simulink model "regulator_lim"  (R2019a)
settings: Solver=FixedStepAuto  StartTime=0.0  StopTime=20  FixedStep=sT  RelTol=1e-3
InitFcn:
  | param;
values from neighbouring files (symbols this model uses):
  A = [0 1; w^2 0]    [continus.m]    (also in discrete.m = [0 1; omega^2 0]; param.m = [0 1; omega^2 0]; param2.m = [0 1; omega^2 0]; param_kf.m)
  B = [0; -w^2]    [continus.m]    (also in discrete.m = [0; -omega^2]; param.m = [0; -omega^2]; param2.m = [0; -omega^2]; param_kf.m)
  C = eye(2)    [discrete.m]    (also in param.m; param2.m; param_kf.m = [w^2 0]; test0.m)
  D = [0 0]'    [discrete.m]    (also in param.m; param2.m; param_kf.m = -w^2; test0.m)
  inix = [0.00 0.0]'    [param.m]    (also in param2.m = [0.05 0.0]'; param_kf.m = [0.0 0.0]')
  iniXzmax = 0.07    [param.m]    (also in param2.m; param_kf.m)
  iniXzmin = -0.07    [param.m]    (also in param2.m; param_kf.m)
  K = [k1 k2]    [continus.m]    (also in discrete.m = -place(A, B, [q1 q2]); param.m; param2.m = dlqr(A,B,Q,H); param_kf.m = -place(A, B, [q1 q2]))
  omega = sqrt(g/zc)    [discrete.m]    (also in param.m; param2.m; test0.m)
  q2 = -0.00005    (= -5e-05)    [discrete.m]    (also in param.m = -0.6; param2.m = -0.5; param_kf.m = -0.5; test0.m = -8-4j)
  sT = 0.01    [discrete.m]    (also in param.m; param2.m; param_kf.m; test0.m)
settings Model: Creator=hideaki  LastModifiedBy=hideaki

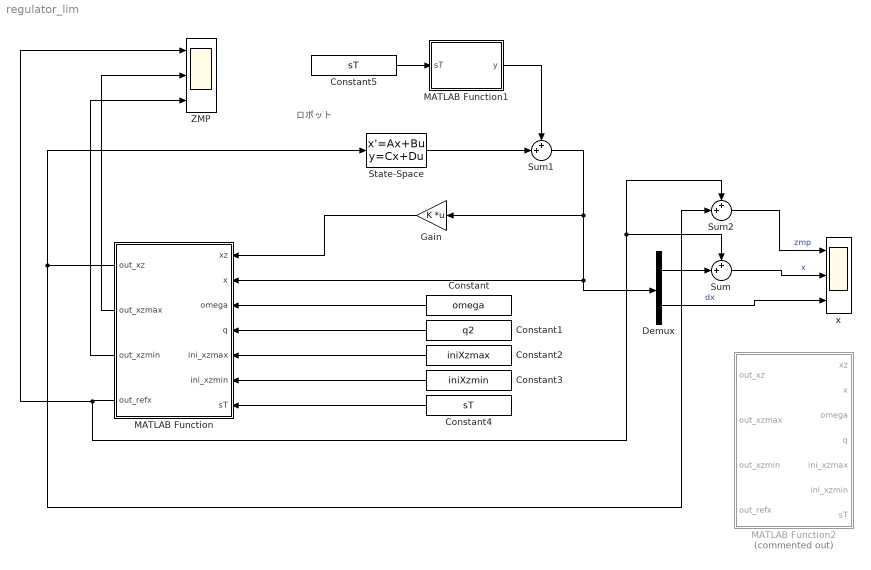
== system regulator_lim ==
  note: ロボット
  Constant : Constant  Value=omega
  Constant1 : Constant  Value=q2
  Constant2 : Constant  Value=iniXzmax
  Constant3 : Constant  Value=iniXzmin
  Constant4 : Constant  Value=sT
  Constant5 : Constant  Value=sT
  Demux : Demux  Outputs=2
  Gain : Gain  Gain=K  Multiplication=Matrix(K*u)
  MATLAB Function : MATLAB Function  TreatAsAtomicUnit=on  SystemSampleTime=sT
  MATLAB Function1 : MATLAB Function  TreatAsAtomicUnit=on
  MATLAB Function2 : MATLAB Function  Commented=on  TreatAsAtomicUnit=on  SystemSampleTime=sT
  State-Space : StateSpace  A=A  B=B  C=C  D=D  InitialCondition=inix
  Sum : Sum  Inputs=++|
  Sum1 : Sum  Inputs=++|
  Sum2 : Sum  Inputs=++|
  ZMP : Scope  NumInputPorts=3
  x : Scope  NumInputPorts=3
  wires:
  Sum1/1 -> Demux/1, MATLAB Function/2(x), Gain/1
  Gain/1 -> MATLAB Function/1(xz)
  MATLAB Function/1(out_xz) -> State-Space/1, Sum2/2
  MATLAB Function/2(out_xzmax) -> ZMP/2
  MATLAB Function/3(out_xzmin) -> ZMP/3
  Constant/1 -> MATLAB Function/3(omega)
  Constant1/1 -> MATLAB Function/4(q)
  Constant2/1 -> MATLAB Function/5(ini_xzmax)
  Constant3/1 -> MATLAB Function/6(ini_xzmin)
  Constant4/1 -> MATLAB Function/7(sT)
  Demux/1 -> Sum/2
  MATLAB Function/4(out_refx) -> ZMP/1, Sum2/1, Sum/1
  Sum/1 -> x/2  "x"
  State-Space/1 -> Sum1/2
  MATLAB Function1/1(y) -> Sum1/1
  Constant5/1 -> MATLAB Function1/1(sT)
  Demux/2 -> x/3  "dx"
  Sum2/1 -> x/1  "zmp"

== matlab function regulator_lim/MATLAB Function1 ==
  data: y output; sT input
function y = nois(sT)
    
    y = zeros(2,1);
    persistent tCnt;
    if isempty(tCnt)
        tCnt = 0;
    end
    
    if (tCnt >= 1 && tCnt <= 1.1) 
        y(2) = -0.4;
    end
    
    tCnt = tCnt + sT;
end

== matlab function regulator_lim/MATLAB Function ==
  data: xz input; out_xz output; x input; out_xzmax output; out_xzmin output; omega input; q input; ini_xzmax input; ini_xzmin input; sT input; out_refx output
%%
% ZMPの出力
% 
%
function [out_xz,out_xzmax,out_xzmin,out_refx] = fcn(xz,x,omega,q,ini_xzmax,ini_xzmin,sT)
    
    persistent tCnt;
    
    %重心の参照位置（目標値）
    persistent refx;
    %実際の支持領域
    persistent xzmax;
    persistent xzmin;
    %refxを基準にした支持領域
    persistent Xzmax;
    persistent Xzmin;
    
    %以下、離床時に計算されて、着地まで保持した後に着地で出力
    persistent s_xz;
    persistent landing;
    persistent s_xzmax;
    persistent s_xzmin;
    persistent s_refx;
    
    %refxを基準にした重心の位置
    X = 0;
    %refxを基準にした重心の速度（速度はどこを基準にしても変わらない）
    dX = 0;
    %refxを基準にしたZMP
    Xz = 0;
    
    if isempty(tCnt)
        tCnt = 0;
        xzmax = ini_xzmax;
        xzmin = ini_xzmin;
        s_xz = xz;
        landing = 0;
        s_xzmax = xzmax;
        s_xzmin = xzmin;
        s_refx = 0;
        refx = getRefx(xzmax,xzmin);
        Xzmax = xzmax - refx;
        Xzmin = xzmin - refx;
    end
    
    X = x(1) - refx;
    dX = x(2);
    Xz = xz -refx;
    
    %立位化安定領域から外れた（xzmin以下）
    if (X+(dX/omega) <= Xzmin) 
        %両足支持
        %支持領域を広げるために、まずは片足支持に移行する
        %if (xzmax == 0.07 && xzmin == -0.07 && landing == 0)
            %強制的に支持領域を狭める（傾いてる方の足を上げる）
            xzmin = 0.01;
            refx = getRefx(xzmax,xzmin);
            %実際のZMP
            s_xz = Xz +refx; 
            %両足支持の場合は離床なのですぐに反映する
            xz = s_xz;
            
            %重心の参照位置は、この時点では変えない
            refx = 0;
            
            %refxを基準としたZMP
            Xz = (1+q)*(X+(dX/omega));
            Xzmin = Xz;
            s_xzmin = Xzmin + refx;
            s_refx = getRefx(xzmax,s_xzmin);
            %実際のZMP（片足支持の場合は着地までに0.6秒かかる）
            s_xz = Xz + refx;
            %着地まで待ち
            tCnt = 0;
            landing = 1;
        %end
    end
    
    %着地
    if (tCnt >= 0.6 && landing == 1) 
        xzmin = s_xzmin;
        refx = s_refx;
        xz = s_xz;
        landing = 2;
    %elseif (landing == 1)
        %実際のロボットでは、ここで両足の中心を重心の参照位置にする（ロボットの遊脚は毎時刻動いている）
        %refx = refx - (abs(s_xzmin) + abs(xzmax))/0.6;
        
    end
    
    
    
    %支持領域の拘束
    if (xz > xzmax) 
        out_xz = xzmax;      
    elseif (xz < xzmin)
        out_xz = xzmin;   
    else
        out_xz = xz;
    end
    
    out_xzmax = xzmax;
    out_xzmin = xzmin;
    out_refx = refx;
    
    tCnt = tCnt + sT;
end

%%
% 重心の参照位置
%
function refx = getRefx(xzmax,xzmin) 
    
    if (0 > xzmax)
        refx = xzmax;
    elseif (0 < xzmin) 
        refx = xzmin;
    else
        refx = (xzmax+xzmin)/2;
    end
    
end

== matlab function regulator_lim/MATLAB Function2 ==
  data: xz input; out_xz output; x input; out_xzmax output; out_xzmin output; omega input; q input; ini_xzmax input; ini_xzmin input; sT input; out_refx output
%%
% ZMPの出力
% 
%
function [out_xz,out_xzmax,out_xzmin,out_refx] = fcn(xz,x,omega,q,ini_xzmax,ini_xzmin,sT)
    
    persistent tCnt;
    
    %重心の参照位置（目標値）
    persistent refx;
    %実際の支持領域
    persistent xzmax;
    persistent xzmin;
    %refxを基準にした支持領域
    persistent Xzmax;
    persistent Xzmin;
    
    %以下、離床時に計算されて、着地まで保持した後に着地で出力
    persistent s_xz;
    persistent landing;
    persistent s_xzmax;
    persistent s_xzmin;
    persistent s_refx;
    
    %refxを基準にした重心の位置
    X = 0;
    %refxを基準にした重心の速度（速度はどこを基準にしても変わらない）
    dX = 0;
    %refxを基準にしたZMP
    Xz = 0;
    
    if isempty(tCnt)
        tCnt = 0;
        xzmax = ini_xzmax;
        xzmin = ini_xzmin;
        s_xz = xz;
        landing = 0;
        s_xzmax = xzmax;
        s_xzmin = xzmin;
        s_refx = 0;
        refx = getRefx(xzmax,xzmin);
        Xzmax = xzmax - refx;
        Xzmin = xzmin - refx;
    end
    
    X = x(1) - refx;
    dX = x(2);
    Xz = xz -refx;
    
    %立位化安定領域から外れた（xzmin以下）
    if (X+(dX/omega) <= Xzmin) 
        %両足支持
        %支持領域を広げるために、まずは片足支持に移行する
        %if (xzmax == 0.07 && xzmin == -0.07 && landing == 0)
            %強制的に支持領域を狭める（傾いてる方の足を上げる）
            xzmin = 0.01;
            refx = getRefx(xzmax,xzmin);
            %実際のZMP
            s_xz = Xz +refx; 
            %両足支持の場合は離床なのですぐに反映する
            xz = s_xz;
            
            %重心の参照位置は、この時点では変えない
            refx = 0;
            
            %refxを基準としたZMP
            Xz = (1+q)*(X+(dX/omega));
            Xzmin = Xz;
            s_xzmin = Xzmin + refx;
            s_refx = getRefx(xzmax,s_xzmin);
            %実際のZMP（片足支持の場合は着地までに0.6秒かかる）
            s_xz = Xz + refx;
            %着地まで待ち
            tCnt = 0;
            landing = 1;
        %end
    end
    
    %着地
    if (tCnt >= 0.6 && landing == 1) 
        xzmin = s_xzmin;
        refx = s_refx;
        xz = s_xz;
        landing = 2;
    elseif (landing == 1)
        %実際のロボットでは、ここで両足の中心を重心の参照位置にする（ロボットの遊脚は毎時刻動いている）
        %refx = refx - (abs(s_xzmin) + abs(xzmax))/0.6;
        
    end
    
    %{
    %立位化安定領域から外れた（xzmin以下）
    if (X+(dX/omega) <= Xzmin) 
        %両足支持
        %支持領域を広げるために、まずは片足支持に移行する
        if (xzmax == 0.07 && xzmin == -0.07)
            %強制的に支持領域を狭める（傾いてる方の足を上げる）
            xzmin = 0.01;
            refx = getRefx(xzmax,xzmin);
            %実際のZMP
            s_xz = Xz +refx; 
            %両足支持の場合は離床なのですぐに反映する
            xz = s_xz;
            landing = 0;
        %片足支持
        elseif (landing == 0)
                
            %refxを基準としたZMP
            Xz = (1-q)*(X+(dX/omega));
            Xzmin = Xz;
            s_xzmin = Xzmin + refx;
            s_refx = getRefx(xzmax,xzmin);
            %実際のZMP（片足支持の場合は着地までに0.6秒かかる）
            s_xz = Xz + refx;
            %着地まで待ち
            tCnt = 0;
            landing = 1;
        end
    end
    
    if (tCnt >= 0.6 && landing == 1) 
        xzmin = s_xzmin;
        refx = s_refx;
        xz = s_xz;
        landing = 2;
    end
    %}
            
    %{
    %着地まで0.6秒と仮定(歩行パターンの1歩にかかる秒数）
    if (tCnt >= 0.6) 
        %立位化安定領域から外れた（xzmin以下）
        if (X+(dX/omega) <= Xzmin) 
            
            %両足支持
            %支持領域を広げるために、まずは片足支持に移行する
            if (xzmax == 0.07 && xzmin == -0.07)
                %強制的に支持領域を狭める（傾いてる方の足を上げる）
                xzmin = 0.01;
                refx = getRefx(xzmax,xzmin);
                %実際のZMP
                xz = Xz +refx; 
                
                %着地まで待ち
                tCnt = 0;
            
            %片足支持
            else
                %refxを基準としたZMP
                Xz = (1-q)*(X+(dX/omega));
                Xzmin = Xz;
                xzmin = Xzmin + refx;
                refx = getRefx(xzmax,xzmin);
                %実際のZMP
                xz = Xz + refx;
            end
        end
        %立位化安定領域から外れた（xzmax以上）
        if (X+(dX/omega) >= xzmax)
            
        end
    end
    %}
    
    %支持領域の拘束
    if (xz > xzmax) 
        out_xz = xzmax;      
    elseif (xz < xzmin)
        out_xz = xzmin;   
    else
        out_xz = xz;
    end
    
    out_xzmax = xzmax;
    out_xzmin = xzmin;
    out_refx = refx;
    
    tCnt = tCnt + sT;
end

%%
% 重心の参照位置
%
function refx = getRefx(xzmax,xzmin) 
    
    if (0 > xzmax)
        refx = xzmax;
    elseif (0 < xzmin) 
        refx = xzmin;
    else
        refx = (xzmax+xzmin)/2;
    end
    
end
